simulink subsystem "BdotController"  (R2021a)
settings: Solver=VariableStepAuto  StartTime=0.0  StopTime=10.0  RelTol=1e-3
undefined symbols (not defined in the file): K_Bdot, Max_magmom, Min_magmom, n
libraries: sharedutil x2, vrlib x1
settings Model: Creator=Laura  LastModifiedBy=Laura

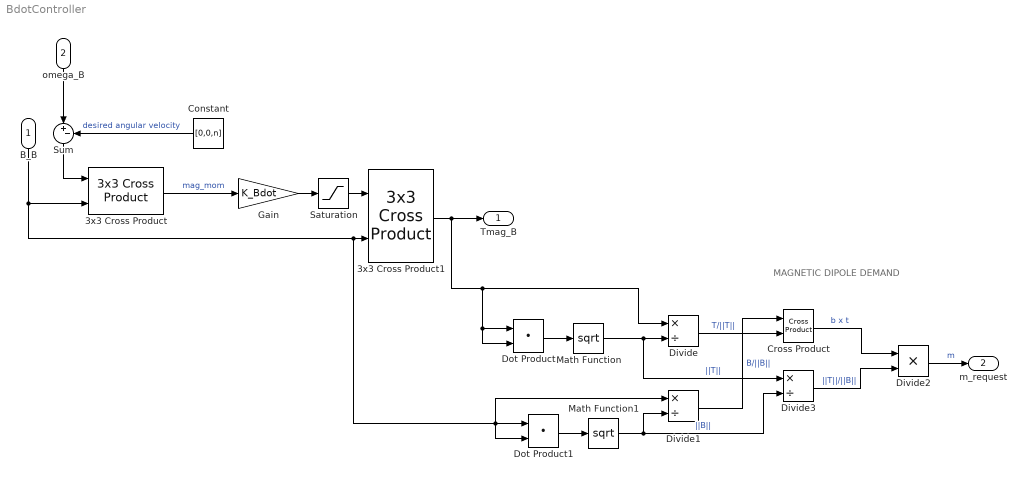
== system BdotController ==
  note: MAGNETIC DIPOLE DEMAND
  B_B : Inport
  omega_B : Inport  Port=2
  3x3 Cross Product : sharedutil/3x3 Cross Product  aMode=aMode
      settings: SourceProductBaseCode=AE,PW,DR,MT,UV,VE
  3x3 Cross Product1 : sharedutil/3x3 Cross Product  aMode=aMode
      settings: SourceProductBaseCode=AE,PW,DR,MT,UV,VE
  Constant : Constant  Value=[0,0,n]
  Cross Product : vrlib/Utilities/Cross Product
  Divide : Product  Inputs=*/
  Divide1 : Product  Inputs=*/
  Divide2 : Product  Inputs=**
  Divide3 : Product  Inputs=*/
  Dot Product : DotProduct  InputSameDT=on  OutDataTypeStr=Inherit: Inherit via internal rule
  Dot Product1 : DotProduct  InputSameDT=on  OutDataTypeStr=Inherit: Inherit via internal rule
  Gain : Gain  Gain=K_Bdot
  Math Function : Math  Operator=sqrt  SignedPower=on  SaturateOnIntegerOverflow=on
  Math Function1 : Math  Operator=sqrt  SignedPower=on  SaturateOnIntegerOverflow=on
  Saturation : Saturate  UpperLimit=Max_magmom  LowerLimit=Min_magmom
  Sum : Sum  Inputs=|+-
  Tmag_B : Outport
  m_request : Outport  Port=2
  wires:
  Gain/1 -> Saturation/1
  3x3 Cross Product/1 -> Gain/1  "mag_mom"
  Sum/1 -> 3x3 Cross Product/1
  omega_B/1 -> Sum/1
  Saturation/1 -> 3x3 Cross Product1/1
  Constant/1 -> Sum/2  "desired angular velocity"
  Divide2/1 -> m_request/1  "m"
  Math Function/1 -> Divide/2, Divide3/1  "||T||"
  Math Function1/1 -> Divide3/2, Divide1/2  "||B||"
  Divide3/1 -> Divide2/2  "||T||/||B||"
  Dot Product1/1 -> Math Function1/1
  Divide1/1 -> Cross Product/1  "B/||B||"
  Cross Product/1 -> Divide2/1  "b x t"
  B_B/1 -> 3x3 Cross Product/2, 3x3 Cross Product1/2, Dot Product1/1, Dot Product1/2, Divide1/1
  Dot Product/1 -> Math Function/1
  3x3 Cross Product1/1 -> Tmag_B/1, Dot Product/2, Dot Product/1, Divide/1
  Divide/1 -> Cross Product/2  "T/||T||"
